simulink model "nav"  (R2025b)
settings: Solver=ode2  StartTime=0.0  StopTime=inf  FixedStep=1/100  RelTol=1e-3
PreLoadFcn:
  | nav_PreLoadFcn
  | stepsize_ctrl = evalin('base', get_param(bdroot, 'FixedStep'));
values from neighbouring files (symbols this model uses):
  navConsts = defineConstants_nav()    [nav_PreLoadFcn.m]
undefined symbols (not defined in the file or in its folder): dspblkCoreblockFVToolHelper, gcbh
libraries: eeGeneralControl x5, simulink x2, sharedutil x1, sharedtransform x1
(part 2 of 2)

== matlab function nav/gps preprocessor ==
  settings: updateMethod=DISCRETE
  data: geodeticReference output Bus: ifr_geodeticReference size=1; hil_on input; parameters input Bus: nav_parameterBus size=1; fixReference input; rawGpsData input Bus: vehicle_gps_position_bus size=1; gps output Bus: ifr_gps size=1; navConsts parameter size=1
function [geodeticReference,gps] =preprocessGps(hil_on,parameters,fixReference,rawGpsData,navConsts)
persistent refPosValid refPosLlhRaw refLlhRawToNed earthMagneticField gravity isInitialized buffer counter
MAX_BUF_SIZE = 200;

if isempty(refPosLlhRaw)
    refPosLlhRaw = int32([navConsts.initialPositionLla(1:2)*1e7; navConsts.initialPositionLla(3)*1e3]);
    refPosValid = false;
    [refLlhRawToNed, earthMagneticField, gravity]=initialize(refPosLlhRaw, single(2020), navConsts);
    isInitialized=false;
    buffer = zeros(MAX_BUF_SIZE,3,'int32'); %Max 40s buffer
    counter = 1;
    %
end

bufferSize = parameters.gpsBufferTime * single(5);
gps.isValid=(rawGpsData.is_valid && rawGpsData.eph<=parameters.gpsAccuracyThreshold);

posLlhRaw=[rawGpsData.lat; rawGpsData.lon; rawGpsData.alt];

if ~isInitialized && gps.isValid
    gpsAvrg = zeros(1,3,'double');
    ctr = 0;
    if ~fixReference
        buffer(counter,:) = [rawGpsData.lat, rawGpsData.lon, rawGpsData.alt]; %update with new values
        if single(mod(counter,MAX_BUF_SIZE)) > bufferSize
            % bufferSize has to be converted from 'real32_T {aka float}' to 'real_T {aka double}' to match other operand of binary expression [-Werror=double-promotion]
            %determine average of gps values as reference
            for i = 0:bufferSize-1 %for loop equals sum(buffer(counter-bufferSize:counter,:))
                ctr = ctr + 1;
                gpsAvrg = gpsAvrg + double(buffer(counter-i,:));
            end
            refPos = int32(gpsAvrg'/ctr);
        else %mod(counter,MAX_BUF_SIZE) <= bufferSize
            %consider all previous elements of buffer matrix
            for i = 1:mod(counter,MAX_BUF_SIZE) %for loop equals sum(buffer(counter-bufferSize:counter,:))
                ctr = ctr + 1;
                gpsAvrg = gpsAvrg + double(buffer(i,:));
            end
            %consider all relevant elements at the end of buffer matrix
            for i = 1:bufferSize-mod(counter,MAX_BUF_SIZE) %for loop equals sum(buffer)'/sum(~all(buffer==0,2))
                currBuff = double(buffer(end+1-i,:));
                if ~isequal(currBuff,zeros(1,3))
                    ctr = ctr + 1;
                    gpsAvrg = gpsAvrg + currBuff;
                end
            end
            refPos = int32(gpsAvrg'/ctr);
        end
        if hil_on && navConsts.airStart %air start in simulation
            refPosLlhRaw=refPos-int32([0*1e7; 0*1e7; navConsts.initialBaroReading*1e3]);
        else
            refPosLlhRaw=refPos;
        end
        if rawGpsData.time_utc_usec~=0
            year=single(1970)+single(rawGpsData.time_utc_usec/(365.24*24*3600*1.0e6));
        else
            year=single(2020);
        end
        [refLlhRawToNed, earthMagneticField, gravity]=initialize(refPosLlhRaw, year, navConsts);
        if counter >= MAX_BUF_SIZE
            counter = 1;
        else
            counter = counter + 1;
        end
    else
        isInitialized=true;
    end
    refPosValid = true;
end

gps.position=refLlhRawToNed.*single(posLlhRaw-[refPosLlhRaw(1:2);0]);
gps.velocity=[rawGpsData.vel_n_m_s; rawGpsData.vel_e_m_s; rawGpsData.vel_d_m_s];

geodeticReference.earthMagneticField = earthMagneticField;
geodeticReference.gravity =            gravity;
geodeticReference.refLlhRawToNed =     refLlhRawToNed;
geodeticReference.refPosLlhRaw =       refPosLlhRaw;
geodeticReference.refPosValid =        refPosValid;
end

function [llhRawToNed, magRefNed, gravity]=initialize(refLlhPosRaw, year, constants)
semiMajorAxis=single(6378137);
eccentricity=single(8.1819190842622e-2);
posScaleFactor=single([1e-7*pi/180; 1e-7*pi/180; 1e-3]);
lattitudeRef=posScaleFactor(1)*single(refLlhPosRaw(1)); %[rad]
longitudeRef=posScaleFactor(2)*single(refLlhPosRaw(2)); %[rad]
heightRef=posScaleFactor(3)*single(refLlhPosRaw(3)); %[m]
R0=semiMajorAxis/sqrt(1-eccentricity^2*sin(lattitudeRef)^2);
llhRawToNed=[(1-eccentricity^2)/semiMajorAxis^2*R0^3+heightRef; (R0+heightRef)*cos(lattitudeRef); -1].*posScaleFactor;

gamma=9.7803253359;
k=0.0019318526464;
dgdh=3.0877e-06;
ldgdh=4.50e-09;
gravity=single([0; 0; gamma*(1+k*sin(lattitudeRef)^2)/sqrt(1-eccentricity^2*sin(lattitudeRef)^2)-(dgdh-ldgdh*sin(lattitudeRef)^2)*heightRef]);
magRefNed=magnet([lattitudeRef; longitudeRef; heightRef], max(single(year-2000), single(0))*365, constants);
end

function magRefNED = magnet(llh, days, constants) % Inputs % r Geocentric radius % theta Latitude measured in degrees positive from equator % phi Longitude measured in degrees positive east from Greenwich % days Decimal days since January 1, 2000 % % Outputs - magnetic field strength in local tangential coordinates % Br B in radial direction % Bt B in theta direction % Bp B in phi direction
lat=pi/2-llh(1);
lon=llh(2);
a=6371200;
r=a+llh(3);
% Checks to see if located at either pole to avoid singularities
if (lat>single(-pi*1e-7) && lat<single(pi*1e-7))
    lat=single(pi*1e-7);
elseif(lat<single(pi*(1+1e-7)) && lat>single(pi*(1-1e-7)))
    lat=single(pi*(1-1e-7));
end

N=13;
g = constants.g0 + constants.dg*days/365.25;
h = constants.h0 + constants.dh*days/365.25;

[Br, Bt, Bp, dP11, dP10, P20, dP20]=deal(single(0));
[P10, P11]=deal(single(1));
[cosLat, sinLat]=deal(cos(lat), sin(lat));
for m=0:N
    for n=1:N
        if m<=n
            % Calculate Legendre polynomials and derivatives recursively
            if n==m
                P2 = sinLat*P11;
                dP2 = sinLat*dP11 + cosLat*P11;
                P11=P2; P10=P11; P20=single(0); dP11=dP2; dP10=dP11; dP20=single(0);
            elseif n==1
                P2 = cosLat*P10;
                dP2 = cosLat*dP10 - sinLat*P10;
                P20=P10; P10=P2; dP20=dP10; dP10=dP2;
            else
                K = ((n-1)^2-m^2)/((2*n-1)*(2*n-3));
                P2 = cosLat*P10 - K*P20;
                dP2 = cosLat*dP10 - sinLat*P10 - K*dP20;
                P20=P10; P10=P2; dP20=dP10; dP10=dP2;
            end
            Br = Br + (a/r)^(n+2)*(n+1)*((g(n,m+1)*cos(m*lon) + h(n,m+1)*sin(m*lon))*P2);
            Bt = Bt + (a/r)^(n+2)*((g(n,m+1)*cos(m*lon) + h(n,m+1)*sin(m*lon))*dP2);
            Bp = Bp + (a/r)^(n+2)*(m*(-g(n,m+1)*sin(m*lon) + h(n,m+1)*cos(m*lon))* P2);
        end
    end
end
magRefSphere = [Br;-Bt;-Bp/sinLat];
e = 0*pi/180;
magRefNED = [-sin(e),-cos(e),0;0,0,1;-cos(e),sin(e),0]*magRefSphere*10^-9;
end

== matlab function nav/imu integration ==
  data: imu input Bus: ifr_imu size=1; translation output single size=6; rotation output single size=4; delayedImu input Bus: ifr_imu size=1; delayedRotation input single size=4; navConsts parameter size=1
function [translation, rotation] = integrateImu(imu, delayedImu, delayedRotation, navConsts)
    persistent quaternion x
    
    delayedImu.acceleration = delayedImu.acceleration;% + [0; 0; 9.81];
    imu.acceleration = imu.acceleration; %+ [0; 0; 9.81];
    dt=navConsts.stepSize;
    n=round(navConsts.filterDelay/dt);
    if isempty(quaternion)
        quaternion=single([1; 0; 0; 0]);
        x=zeros(6, 1, 'single');
    end
    rotation=quaternion;
    translation=x;
    
    I=eye(3, 'single');
    O=zeros(3, 'single');
    x=[I, dt*I; O, I]*x+[single(0.5)*dt^2*I, -dt^2*(n+single(0.5))*I; dt*I, -dt*I]*[quatToMat(rotation)'*imu.acceleration; quatToMat(delayedRotation)'*delayedImu.acceleration];
    quaternion=quaternion+single(0.5)*dt*[-imu.rate'*quaternion(2:4); imu.rate*quaternion(1)-cross(imu.rate, quaternion(2:4))];
    quaternion=quaternion/norm(quaternion);
end

function mat=quatToMat(quat)
    [q0, q1, q2, q3]=deal(quat(1), quat(2), quat(3), quat(4));
    mat=[1-2*(q2^2+q3^2), 2*(q1*q2+q3*q0), 2*(q1*q3-q2*q0); ...
         2*(q1*q2-q3*q0), 1-2*(q1^2+q3^2), 2*(q2*q3+q1*q0); ...
         2*(q1*q3+q2*q0), 2*(q2*q3-q1*q0), 1-2*(q1^2+q2^2)];
end

== matlab function nav/imu preprocessor ==
  settings: updateMethod=DISCRETE
  data: time input single size=1; gyroBiasOut output; parameters input Bus: nav_parameterBus; fixGyroBias input boolean size=1; rateRaw input single size=3; imu output Bus: ifr_imu size=1; accRaw input single size=3
function [gyroBiasOut,imu]=preprocessImuData(time,parameters,fixGyroBias,rateRaw,accRaw)
persistent gyroBias fixed
if isempty(gyroBias)
    gyroBias=zeros(3, 1, 'single');
    fixed=false;
end

if ~fixGyroBias && ~fixed
    if isequal(parameters.imu_filt.use_rte,single(1)) %IMU filter module already uses gyro bias signal
        gyroBias=gyroBias+parameters.biasSmoothingGain*(rateRaw-gyroBias);
    end
else
    fixed=true;
end
imu.time=time;
imu.rate=rateRaw-gyroBias;
%imu.rate=rateRaw;
imu.acceleration= accRaw;
gyroBiasOut=gyroBias;
end

== matlab function nav/Actuator Model/limit control output3 ==
  data: u input single; y output single
function y = control_output_sat(u)

y = zeros(size(u),'single');
y(:) = min(max(u(:),0),1);

end

== matlab function nav/magnetometer preprocessor ==
  data: vehicle_mag input Bus: vehicle_magnetometer_bus; mag output Bus: ifr_mag size=1
function mag=preprocessMagnetometer(vehicle_mag)
    mag.isValid=vehicle_mag.is_valid;
    mag.magneticField=1000.0*vehicle_mag.magnetometer_ga;
                                %single*(1e-4)
end

== matlab function nav/Subsystem1/MATLAB Function ==
  data: u input; y output uint8
function y = fcn(u)
% assign rc-modes depending on the switch position
if u < single(-0.33) %test_controls
    y = uint8(1);
elseif u < single(0.33) %steady_state
    y = uint8(2);
else %wp_tracking
    y = uint8(3);
end

== matlab function nav/navigation filter ==
  data: imu input Bus: ifr_imu size=1; z_valid output; para input Bus: nav_parameterBus size=1; pos output single size=3; baro input Bus: ifr_baro size=1; geoRef input Bus: ifr_geodeticReference; gps input Bus: ifr_gps size=1; mag input Bus: ifr_mag size=1; startFilter input boolean size=1; vel output single size=3; att output single size=4; navConsts parameter size=1; errVar output single size=9; sensors_valid output; mag_logger output Bus: navigation_mag_bus
function [z_valid,pos,vel,att,errVar,sensors_valid,mag_logger]=estimateVehicleState(imu,para,baro,geoRef,gps,mag,startFilter,navConsts)
persistent state covariance filterIsRunning timing

if isempty(state)
    state=[zeros(6, 1, 'single'); 1; zeros(3, 1, 'single')];
    covariance=diag(single([25, 25, 25, 4, 4, 4, 0.1, 0.1, 0.1]));
    filterIsRunning=false;
    timing=struct('sinceGps', para.gpsTimeout, 'lastTime', imu.time-navConsts.stepSize);
end

stepSize=imu.time-timing.lastTime;
timing.lastTime=imu.time;

if gps.isValid
    if timing.sinceGps>=para.gpsTimeout && filterIsRunning
        [state, covariance]=resetUsingGps(para, state, covariance, gps);
        gps.isValid=false;
    end
    timing.sinceGps=single(0);
else
    timing.sinceGps=timing.sinceGps+stepSize;
end

z_valid = timing.sinceGps<para.gpsTimeout;

if ~filterIsRunning
    if startFilter
        state(7:10)=initQuat(mag.magneticField, imu.acceleration);
        covariance(7:9, 7:9)=diag(single([0.1,0.1,0.1]));
        % next time GPS is available, horizontal position and velocity
        % shall be set to measurement rather than being updated
        [timing.sinceGps, filterIsRunning]=deal(para.gpsTimeout, true);
    end
    [pos, vel, att, errVar]=deal(state(1:3), state(4:6), state(7:10), diag(covariance));
    mag_logger.is_valid = false;
    mag_logger.state = zeros(10, 1, 'single');
    mag_logger.meas = zeros(3, 1, 'single');
    mag_logger.t = zeros(9, 1, 'single');
    mag_logger.ref = zeros(3, 1, 'single');
    mag_logger.residual = zeros(1, 1, 'single');
    mag_logger.h = zeros(9, 1, 'single');
    mag_logger.r = zeros(1, 1, 'single');
    mag_logger.gibbs_state = zeros(9, 1, 'single');
    mag_logger.attitude = zeros(3, 1, 'single');
else
    if timing.sinceGps<para.gpsTimeout
        [pos, vel, att, errVar, state, covariance, mag_logger]=runFilter(para, state, covariance, 1:9,...
            imu, stepSize, mag, gps, baro,geoRef);
    else
        [pos, vel, att, errVar, state, covariance, mag_logger]=runFilter(para, state, covariance, [3, 6:9],...
            imu, stepSize, mag, gps, baro,geoRef);
    end
end
sensors_valid = [mag.isValid;gps.isValid;baro.isValid];
end

function [position, velocity, attitude, errorVariances, state, covariance, mag_logger]=runFilter(parameters, state, covariance, subStateIndices, imu, stepSize,...
    mag, gps, baro,geoRef)
[state, covariance, mag_logger]=update(parameters, state, covariance, subStateIndices, mag, gps, baro, imu.acceleration,geoRef);
[position, velocity, attitude, errorVariances]=deal(state(1:3), state(4:6), state(7:10), diag(covariance));
[state, covariance]=predict(parameters, state, covariance, subStateIndices, imu, stepSize,geoRef.gravity);
end

function [state, covariance]=predict(parameters, state, covariance, iSub, imu, stepSize, g)
[v, q]=deal(state(4:6), state(7:10));

I=eye(3, 'single');
O=zeros(3, 'single');

bodyToGeo=quatToMat(q)';
stateIncrement=[stepSize*v+0.5*stepSize^2*(bodyToGeo*imu.acceleration+g);...
    stepSize*(bodyToGeo*imu.acceleration+g);...
    0.5*stepSize*[0, -imu.rate'; imu.rate, -skew(imu.rate)]*q];
F=[I, stepSize*I, -0.5*stepSize^2*bodyToGeo*skew(imu.acceleration);...
    O,          I,       -stepSize*bodyToGeo*skew(imu.acceleration);...
    O,          O,                        I-stepSize*skew(imu.rate)];
GQImuGT=[0.25*stepSize^4*parameters.sigmaAcc^2*I, 0.5*stepSize^3*parameters.sigmaAcc^2*I,                                         O;...
    0.5*stepSize^3*parameters.sigmaAcc^2*I,     stepSize^2*parameters.sigmaAcc^2*I,                                         O;...
    O,                                            O, stepSize^2*parameters.sigmaGyro^2*I];

covariance(iSub, iSub)=F(iSub, iSub)*covariance(iSub, iSub)*F(iSub, iSub)'+GQImuGT(iSub, iSub);
state([iSub, end])=state([iSub, end])+stateIncrement([iSub, end]);
state(7:10)=normalize(state(7:10));
end

function [state, covariance, mag_logger]=update(parameters, state, covariance, iSub, mag, gps, baro, acc, geoRef)
geoToBody=quatToMat(state(7:10));
bodyToGeo=geoToBody';
gibbsState=[state(1:6); zeros(3, 1, 'single')]; % expected attitude error (gibbs vector) is zero
if mag.isValid
    [residual_mag, H, R]=magMeasurementModel(parameters, mag.magneticField, bodyToGeo,geoRef.earthMagneticField);
    [gibbsState(iSub), covariance(iSub, iSub)]=performKalmanUpdate(gibbsState(iSub), covariance(iSub, iSub), residual_mag, H(:, iSub), R);
    mag_logger.is_valid = true;
    mag_logger.state = state;
    mag_logger.meas = mag.magneticField;
    mag_logger.t = reshape(bodyToGeo, [9 1]);
    mag_logger.ref = geoRef.earthMagneticField;
    mag_logger.residual = residual_mag;
    mag_logger.h = H';
    mag_logger.r = R;
    mag_logger.gibbs_state = gibbsState;
    mag_logger.attitude = zeros(3, 1, 'single');
else
    mag_logger.is_valid = false;
    mag_logger.state = zeros(10, 1, 'single');
    mag_logger.meas = zeros(3, 1, 'single');
    mag_logger.t = zeros(9, 1, 'single');
    mag_logger.ref = zeros(3, 1, 'single');
    mag_logger.residual = zeros(1, 1, 'single');
    mag_logger.h = zeros(9, 1, 'single');
    mag_logger.r = zeros(1, 1, 'single');
    mag_logger.gibbs_state = gibbsState;
    mag_logger.attitude = zeros(3, 1, 'single');
end
if gps.isValid
    [residual, H, R]=gpsMeasurementModel(parameters, gps.position, gps.velocity, gibbsState(1:3), gibbsState(4:6), geoRef.refPosLlhRaw);
    [gibbsState(iSub), covariance(iSub, iSub)]=performKalmanUpdate(gibbsState(iSub), covariance(iSub, iSub), residual, H(:, iSub), R);
elseif numel(iSub)<numel(gibbsState)-2 % only use acceleration update if neither GPS nor LOS rate are available
    [residual, H, R]=accMeasurementModel(parameters, acc, geoToBody, geoRef.gravity);
    [gibbsState(iSub), covariance(iSub, iSub)]=performKalmanUpdate(gibbsState(iSub), covariance(iSub, iSub), residual, H(:, iSub), R);
    gibbsState(4:5)=0.995*gibbsState(4:5); % velocity estimate is likely to be far off, hence it is damped
end
if baro.isValid
    [residual, H, R]=baroMeasurementModel(parameters, baro.height, -gibbsState(3));
    [gibbsState(iSub), covariance(iSub, iSub)]=performKalmanUpdate(gibbsState(iSub), covariance(iSub, iSub), residual, H(:, iSub), R);
end
state=[gibbsState(1:6); normalize(quaternionProduct(state(7:10), [2; gibbsState(7:9)]))];
end

function [residual_mag, measurementMatrix, measurementCovariance]=magMeasurementModel(parameters, mag, bodyToGeo, magGeoRef)
magGeo=bodyToGeo*mag;
measurementMatrix=[zeros(1, 6, 'single'), bodyToGeo(3, :)];
normProduct=norm(magGeoRef(1:2))*norm(magGeo(1:2));
denominator=normProduct+magGeoRef(1:2)'*magGeo(1:2);
epsilon=single(1e-3);
sigmaMag=single(1e-4)*parameters.sigmaMag; % unit should be T but is Gs
if denominator>epsilon*normProduct
    residual_mag=2*(magGeo(1)*magGeoRef(2)-magGeo(2)*magGeoRef(1))/denominator;
    measurementCovariance=(2*norm(magGeo(1:2))*sigmaMag/denominator)^2;
else % error is close to 180 deg, circumventing singularity...
    residual_mag=2*sqrt(2/epsilon-1);
    measurementCovariance=(2*sigmaMag/(epsilon*norm(magGeoRef(1:2))))^2;
end
end

function [residual, measurementMatrix, measurementCovariance]=gpsMeasurementModel(parameters, gpsPos, gpsVel, pos, vel, geoRef)
residual=[gpsPos-pos; gpsVel-vel];
measurementMatrix=[eye(6, 'single'), zeros(6, 3, 'single')];
measurementCovariance=diag([parameters.sigmaGpsPosXy*[1/cos(pi/180*1e-7*double(geoRef(1))); 1]; parameters.sigmaGpsPosZ;...
    parameters.sigmaGpsVelXy*[1/cos(pi/180*1e-7*double(geoRef(1))); 1]; parameters.sigmaGpsVelZ].^2);
end

function [residual, measurementMatrix, measurementCovariance]=baroMeasurementModel(parameters, baroHeight, height)
residual=baroHeight-height;
measurementMatrix=[zeros(1, 2, 'single'), -1, zeros(1, 6, 'single')];
measurementCovariance=parameters.sigmaBaro^2;
end

function [residual, measurementMatrix, measurementCovariance]=accMeasurementModel(parameters, acc, geoToBody, gravity)
residual=acc+geoToBody*gravity;
measurementMatrix=[zeros(3, 6, 'single'), -skew(geoToBody*gravity)];
measurementCovariance=parameters.sigmaAccelerationUpdate^2*eye(3, 'single');
end

function [state, covariance]=performKalmanUpdate(state, covariance, residual, H, R)
S=H*covariance*H'+R;
K=covariance*H'/S;
state=state+K*residual;
covariance=covariance-K*H*covariance;
end

function [state, covariance]=resetUsingGps(parameters, state, covariance, gps)
state(1:2)=gps.position(1:2);
covariance(1:2, 1:2)=parameters.sigmaGpsPosXy.^2*eye(2, 'single');
[covariance(1:2, 3:end), covariance(3:end, 1:2)]=deal(single(0));
state(4:6)=gps.velocity;
covariance(4:6, 4:6)=diag([parameters.sigmaGpsVelXy([1; 1]); parameters.sigmaGpsVelZ].^2);
[covariance(4:6, [1:3, 7:end]), covariance([1:3, 7:end], 4:6)]=deal(single(0));
end

function q=initQuat(magMeas, accMeas)
% geodetic axes in body frame using Gram-Schmidt process
basisZ=-normalize(accMeas);
basisX=normalize(magMeas-(magMeas'*basisZ)*basisZ);
q=matToQuat([basisX, cross(basisZ, basisX), basisZ]);
end

function n=normalize(v)
n=v./repmat(sqrt(sum(v.^2)), size(v, 1), 1);
end

function s=skew(v)
s=[     0, -v(3),  v(2);...
    v(3),     0, -v(1);...
    -v(2),  v(1),     0];
end

function prod=quaternionProduct(q, p)
[q0, qVec, p0, pVec]=deal(q(1), q(2:4), p(1), p(2:4));
prod=[q0*p0-qVec'*pVec; q0*pVec+p0*qVec+cross(qVec, pVec)];
end

function mat=quatToMat(quat)
[q0, q1, q2, q3]=deal(quat(1), quat(2), quat(3), quat(4));
mat=[1-2*(q2^2+q3^2), 2*(q1*q2+q3*q0), 2*(q1*q3-q2*q0); ...
    2*(q1*q2-q3*q0), 1-2*(q1^2+q3^2), 2*(q2*q3+q1*q0); ...
    2*(q1*q3+q2*q0), 2*(q2*q3-q1*q0), 1-2*(q1^2+q2^2)];
end

function quat=matToQuat(mat)
quat=zeros(4, 1, 'single');
tr=trace(mat);
if (tr>0)
    quat=[1+tr; mat(2, 3)-mat(3, 2); mat(3, 1)-mat(1, 3); mat(1, 2)-mat(2, 1)];
else
    [~, iMaxD]=max(diag(mat));
    switch iMaxD
        case 1, quat=[mat(2, 3)-mat(3, 2); 1+mat(1, 1)-mat(2, 2)-mat(3, 3); mat(1, 2)+mat(2, 1); mat(3, 1)+mat(1, 3)];
        case 2, quat=[mat(3, 1)-mat(1, 3); mat(1, 2)+mat(2, 1); 1-mat(1, 1)+mat(2, 2)-mat(3, 3); mat(2, 3)+mat(3, 2)];
        case 3, quat=[mat(1, 2)-mat(2, 1); mat(3, 1)+mat(1, 3); mat(2, 3)+mat(3, 2); 1-mat(1, 1)-mat(2, 2)+mat(3, 3)];
    end
end
quat=normalize(quat);
end

== matlab function nav/MATLAB Function1 ==
  data: baro_rel input Bus: ifr_baro; h_ref input; ref_pos input; ref_valid input; baro_abs output Bus: ifr_baro
function baro_abs  = fcn(baro_rel,h_ref,ref_pos,ref_valid)

baro_abs.isValid = baro_rel.isValid;

if ref_valid
    baro_abs.height  = baro_rel.height + single(ref_pos(3)*1e-3);
else
    baro_abs.height  = baro_rel.height + h_ref;
end

end

== matlab function nav/MATLAB Function2 ==
  data: attitude input; mag_logger input Bus: navigation_mag_bus; mag_logger output
function mag_logger = fcn(attitude, mag_logger)

mag_logger.attitude = attitude;

== matlab function nav/MATLAB Function5 ==
  data: accel input; aero_est output; navConsts parameter
function aero_est = anglesEstimation(accel,navConsts)
aero_est = [(accel(3)+navConsts.g)/navConsts.Zalpha;accel(2)/navConsts.Ybeta];

== matlab function nav/vehicle_state_bus_creator/Angles Estimation ==
  data: speeds output single size=2; euler input single size=3; vel input single size=3; Va input; param input Bus: nav_parameterBus; track output single size=2
function [speeds,track] = anglesEstimation(euler,vel,Va,param)

Vk = norm(vel);
if isnan(Va) || Va < single(2)
    Va = single(2);
end
if isnan(Vk)
    Vk = single(0);
end

if Vk > param.chiVel
    chi = atan2(vel(2), vel(1));
    gamma = asin(-vel(3)/norm(vel));
    V_A   = Va;
else
    chi = euler(3); % psi
    gamma = single(0); %attitude(2); %theta
    V_A   = Vk;
end

if param.VaDisabled
    V_A   = Vk;
end

track = [gamma, chi]';
speeds = [Vk, V_A]';
end

== matlab function nav/MATLAB Function ==
  data: quat input; eul_rad output
function eul_rad=quat2euler(quat)

eul_rad = single([0;0;0]);
ysqr = quat(3) * quat(3);

t0 = 2 * (quat(1) * quat(2) + quat(3) * quat(4));
t1 = 1 - 2 * (quat(2) * quat(2) + ysqr);
eul_rad(1) = atan2(t0, t1);

t2 = 2 * (quat(1) * quat(3) - quat(4) * quat(2));
if t2 > 1
    t2 = single(1);
elseif t2 < -1
    t2 = -single(1);
end
eul_rad(2) = asin(t2);

t3 = 2 * (quat(1) * quat(4) + quat(2) * quat(3));
t4 = 1 - 2 * (ysqr + quat(4) * quat(4));
eul_rad(3) = atan2(t3, t4);

end

== matlab function nav/Actuator Model/MATLAB Function1 ==
  data: in input; out output
function out = fcn(in)

out = [in(1:3);0.5*in(4)+0.5]; %scale thrust from [-1,1] to [0,1]
